simulink model "lorenz"  (R2024a)
settings: Solver=VariableStepAuto  StartTime=0.0  StopTime=10  MinStep=1e-3  RelTol=1e-4
settings Model: Creator=perruquetti  LastModifiedBy=perruquetti

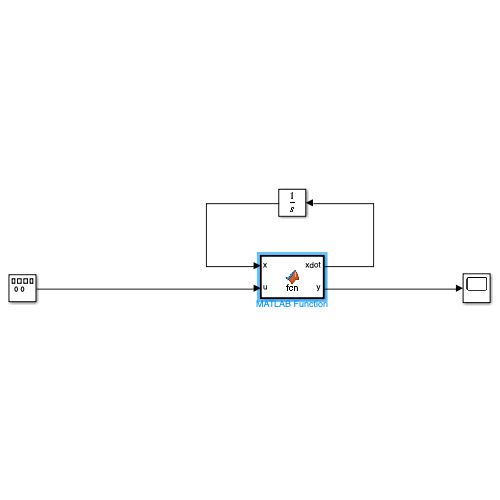
[thumbnail: Simulink's stored preview of the top-level diagram]
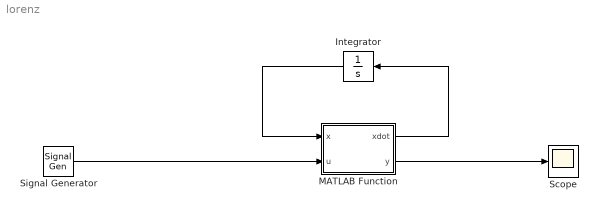
== system lorenz ==
  Integrator : Integrator  InitialCondition="[0.012;  0; 0.84]"
  MATLAB Function : MATLAB Function  TreatAsAtomicUnit=on
  Scope : Scope
  Signal Generator : SignalGenerator  Amplitude=0.1  Units=rad/sec
  wires:
  MATLAB Function/1(xdot) -> Integrator/1
  Integrator/1 -> MATLAB Function/1(x)
  MATLAB Function/2(y) -> Scope/1
  Signal Generator/1 -> MATLAB Function/2(u)

== matlab function lorenz/MATLAB Function ==
  data: x input; xdot output; u input; y output
function [xdot,y] = fcn(x,u)
% constants
    sigma = 10; 
    b = 8/3;
    rho = 28;
% nonlinear set of equations
    xdot = [sigma*(x(2)-x(1));
        rho*x(1)-x(2)-x(1)*x(3);
        x(1)*x(2)-b*x(3)+0.1*u];
    y = x';
